simulink model "Gaussian_Distribution_validation"  (R2024a)
settings: Solver=VariableStepAuto  StartTime=0.0  StopTime=0.005  RelTol=1e-3
libraries: hdlBasic x26, vmcUtilities x1
settings Model: Creator=ehtisham  LastModifiedBy=ehtisham

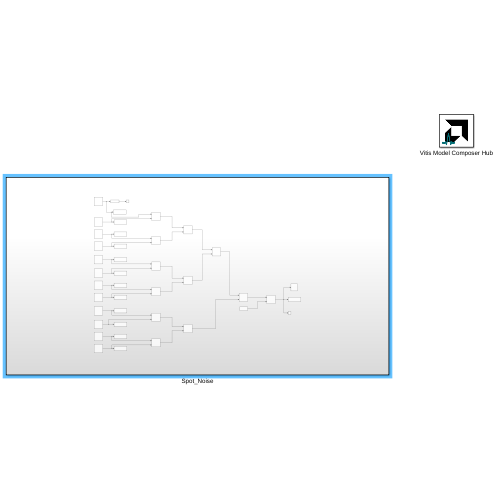
[thumbnail: Simulink's stored preview of the top-level diagram]
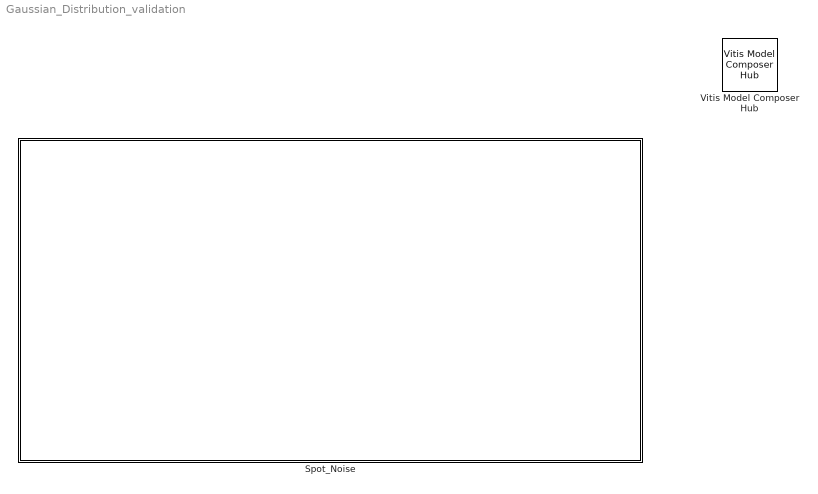
== system Gaussian_Distribution_validation ==
  Spot_Noise : Subsystem
  Vitis Model Composer Hub : vmcUtilities/Vitis Model Composer Hub  Tag=genX  CodeGeneration=off  SubsystemName=Spot_Noise  CompilationType=HDLCompilation  ExportTypeV2=IP Catalog  StartColumn=1  NumberOfColumns=1  TargetDirectory=./netlist  exportDesign=off  analyzeDesign=off  validateDesignOnHw=off  ExportType=AI Engines  IpVendor=xilinx.com  IpLibrary=hls  IpVersion=1.0  IpHWLanguage=Verilog  AieCompilerOptions={}  AieSimulatorOptions={}  CreateTestbench=off  TestbenchStackSize=10  RunRtlSim=off  RunCSim=off  RunAieSim=off  AieSimTimeout=50000  RunAieSimProfiling=off  LaunchVitisAnalyzer=off  PlotOutput=off  RunX86Sim=off  X86SimTimeout=10  GenHwImage=off  GenLibadfXo=on  GenHwValidationCode=off  PlatformType=Not Specified  HwSystemType=Baremetal  HwValidationTarget=hw  ProjDevice=Zynq UltraScale+ ZCU102 Evaluation Board (xczu9eg-ffvb1156-2-e)  ProjDevicePart=xczu9eg-ffvb1156-2-e  AIEType=None  SamplePeriod=-1  ClockFrequency=200  DataPathParallelism=1  xilinxfamily=zynquplus  part=xczu9eg  speed=-2-e  package=ffvb1156  directory=./netlist/ip/Spot_Noise/src  testbench=off  incr_netlist=off  synthesis_tool=Vivado  clock_wrapper=Clock Enables  dbl_ovrd=According to Block Masks  dcm_input_clock_period=10  sysclk_period=4  simulink_period=1/245760000  eval_field=0  LogFileName=''  NThreads=4

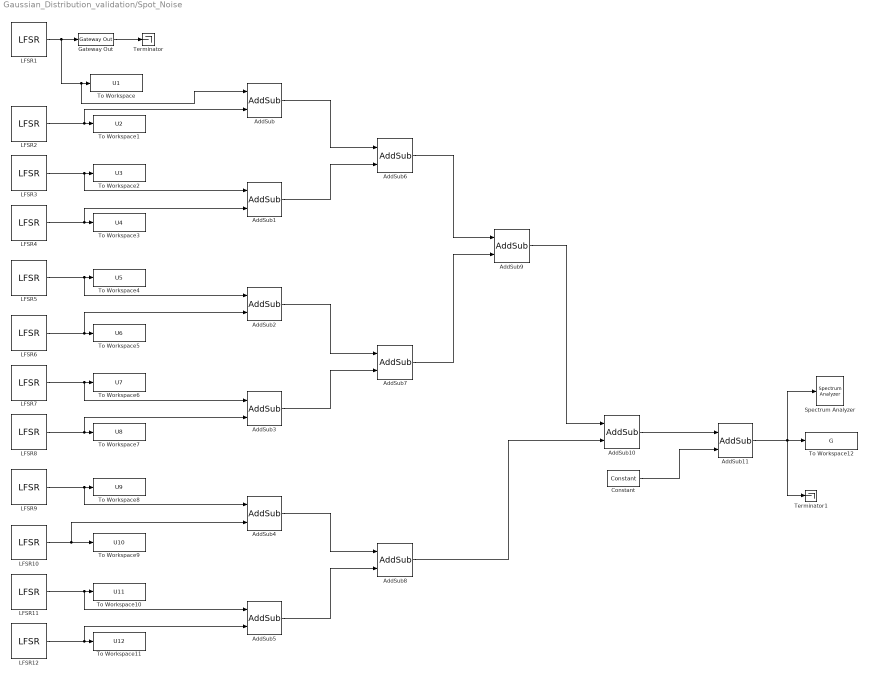
== system Gaussian_Distribution_validation/Spot_Noise ==
  AddSub{,1..10} (11 alike) : hdlBasic/AddSub  mode=Addition  use_carryin=off  use_carryout=off  en=off  latency=0  precision=Full  arith_type=Unsigned  n_bits=16  bin_pt=14  quantization=Truncate  overflow=Wrap  use_behavioral_HDL=off  hw_selection=Fabric  pipelined=off  XmcBlockStatus=1  maskContainerNames=tabcontainer1  block_type=addsub  block_config=sysgen:Addsub_config
  AddSub11 : hdlBasic/AddSub  mode=Subtraction  use_carryin=off  use_carryout=off  en=off  latency=0  precision=Full  arith_type=Unsigned  n_bits=16  bin_pt=14  quantization=Truncate  overflow=Wrap  use_behavioral_HDL=off  hw_selection=Fabric  pipelined=off  XmcBlockStatus=1  maskContainerNames=tabcontainer1  block_type=addsub  block_config=sysgen:Addsub_config
  Constant : hdlBasic/Constant  const=6  gui_display_data_type=Fixed-point  arith_type=Unsigned  n_bits=3  bin_pt=0  preci_type=Single  exp_width=8  frac_width=24  explicit_period=off  period=1  XmcBlockStatus=1  maskContainerNames=tabcontainer1  block_type=constant  block_config=sysgen:Constant_config
  Gateway Out : hdlBasic/Gateway Out  inherit_from_input=off  hdl_port=on  rows=1  columns=1  UseAsDAC=off  DACChannel='1'  interface=None  automatic_assignment=on  address_offset=hex2dec('00')  intf_name=''  intf_description=''  timing_constraint=None  locs_specified=off  LOCs={}  io_standard={}  XmcBlockStatus=1  maskContainerNames=group4  block_type=gatewayout  block_config=sysgen:gateway_out_config  block_width_w=590  block_height_w=620  block_width=620  block_height=750
  LFSR1 : hdlBasic/LFSR  lfsr_type=Fibonacci  gate_type=XNOR  n_bits=16  maxpolynomial=off  polynomial='2D'  rst_value='1'  rst=off  en=off  reloadable_seed=off  input_type=off  output_type=on  arith_type=Unsigned  bin_pt=16  explicit_period=on  period=1/245760000  XmcBlockStatus=1  maskContainerNames=tabcontainer1  block_type=lfsr  block_config=sysgen:LFSR_config
  LFSR10 : hdlBasic/LFSR  lfsr_type=Fibonacci  gate_type=XNOR  n_bits=16  maxpolynomial=off  polynomial='15D'  rst_value='1'  rst=off  en=off  reloadable_seed=off  input_type=off  output_type=on  arith_type=Unsigned  bin_pt=16  explicit_period=on  period=1/245760000  XmcBlockStatus=1  maskContainerNames=tabcontainer1  block_type=lfsr  block_config=sysgen:LFSR_config
  LFSR11 : hdlBasic/LFSR  lfsr_type=Fibonacci  gate_type=XNOR  n_bits=16  maxpolynomial=off  polynomial='197'  rst_value='1'  rst=off  en=off  reloadable_seed=off  input_type=off  output_type=on  arith_type=Unsigned  bin_pt=16  explicit_period=on  period=1/245760000  XmcBlockStatus=1  maskContainerNames=tabcontainer1  block_type=lfsr  block_config=sysgen:LFSR_config
  LFSR12 : hdlBasic/LFSR  lfsr_type=Fibonacci  gate_type=XNOR  n_bits=16  maxpolynomial=off  polynomial='1A1'  rst_value='1'  rst=off  en=off  reloadable_seed=off  input_type=off  output_type=on  arith_type=Unsigned  bin_pt=16  explicit_period=on  period=1/245760000  XmcBlockStatus=1  maskContainerNames=tabcontainer1  block_type=lfsr  block_config=sysgen:LFSR_config
  LFSR2 : hdlBasic/LFSR  lfsr_type=Fibonacci  gate_type=XNOR  n_bits=16  maxpolynomial=off  polynomial='39'  rst_value='1'  rst=off  en=off  reloadable_seed=off  input_type=off  output_type=on  arith_type=Unsigned  bin_pt=16  explicit_period=on  period=1/245760000  XmcBlockStatus=1  maskContainerNames=tabcontainer1  block_type=lfsr  block_config=sysgen:LFSR_config
  LFSR3 : hdlBasic/LFSR  lfsr_type=Fibonacci  gate_type=XNOR  n_bits=16  maxpolynomial=off  polynomial='3F'  rst_value='1'  rst=off  en=off  reloadable_seed=off  input_type=off  output_type=on  arith_type=Unsigned  bin_pt=16  explicit_period=on  period=1/245760000  XmcBlockStatus=1  maskContainerNames=tabcontainer1  block_type=lfsr  block_config=sysgen:LFSR_config
  LFSR4 : hdlBasic/LFSR  lfsr_type=Fibonacci  gate_type=XNOR  n_bits=16  maxpolynomial=off  polynomial='53'  rst_value='1'  rst=off  en=off  reloadable_seed=off  input_type=off  output_type=on  arith_type=Unsigned  bin_pt=16  explicit_period=on  period=1/245760000  XmcBlockStatus=1  maskContainerNames=tabcontainer1  block_type=lfsr  block_config=sysgen:LFSR_config
  LFSR5 : hdlBasic/LFSR  lfsr_type=Fibonacci  gate_type=XNOR  n_bits=16  maxpolynomial=off  polynomial='BD'  rst_value='1'  rst=off  en=off  reloadable_seed=off  input_type=off  output_type=on  arith_type=Unsigned  bin_pt=16  explicit_period=on  period=1/245760000  XmcBlockStatus=1  maskContainerNames=tabcontainer1  block_type=lfsr  block_config=sysgen:LFSR_config
  LFSR6 : hdlBasic/LFSR  lfsr_type=Fibonacci  gate_type=XNOR  n_bits=16  maxpolynomial=off  polynomial='D7'  rst_value='1'  rst=off  en=off  reloadable_seed=off  input_type=off  output_type=on  arith_type=Unsigned  bin_pt=16  explicit_period=on  period=1/245760000  XmcBlockStatus=1  maskContainerNames=tabcontainer1  block_type=lfsr  block_config=sysgen:LFSR_config
  LFSR7 : hdlBasic/LFSR  lfsr_type=Fibonacci  gate_type=XNOR  n_bits=16  maxpolynomial=off  polynomial='12F'  rst_value='1'  rst=off  en=off  reloadable_seed=off  input_type=off  output_type=on  arith_type=Unsigned  bin_pt=16  explicit_period=on  period=1/245760000  XmcBlockStatus=1  maskContainerNames=tabcontainer1  block_type=lfsr  block_config=sysgen:LFSR_config
  LFSR8 : hdlBasic/LFSR  lfsr_type=Fibonacci  gate_type=XNOR  n_bits=16  maxpolynomial=off  polynomial='13D'  rst_value='1'  rst=off  en=off  reloadable_seed=off  input_type=off  output_type=on  arith_type=Unsigned  bin_pt=16  explicit_period=on  period=1/245760000  XmcBlockStatus=1  maskContainerNames=tabcontainer1  block_type=lfsr  block_config=sysgen:LFSR_config
  LFSR9 : hdlBasic/LFSR  lfsr_type=Fibonacci  gate_type=XNOR  n_bits=16  maxpolynomial=off  polynomial='14F'  rst_value='1'  rst=off  en=off  reloadable_seed=off  input_type=off  output_type=on  arith_type=Unsigned  bin_pt=16  explicit_period=on  period=1/245760000  XmcBlockStatus=1  maskContainerNames=tabcontainer1  block_type=lfsr  block_config=sysgen:LFSR_config
  Spectrum Analyzer : SpectrumAnalyzer  WindowPosition=[365.000000,160.000000,800.000000,500.000000,]  ScopeFrameLocation=window  Span=245760000  StartFrequency=-122880000  StopFrequency=122880000  YLimits=[-9.5999377,7.8120668]
  Terminator : Terminator
  Terminator1 : Terminator
  To Workspace : ToWorkspace  VariableName=U1  SaveFormat=Timeseries  SampleTime=-1
  To Workspace1 : ToWorkspace  VariableName=U2  SaveFormat=Timeseries  SampleTime=-1
  To Workspace10 : ToWorkspace  VariableName=U11  SaveFormat=Timeseries  SampleTime=-1
  To Workspace11 : ToWorkspace  VariableName=U12  SaveFormat=Timeseries  SampleTime=-1
  To Workspace12 : ToWorkspace  VariableName=G  SaveFormat=Timeseries  SampleTime=-1
  To Workspace2 : ToWorkspace  VariableName=U3  SaveFormat=Timeseries  SampleTime=-1
  To Workspace3 : ToWorkspace  VariableName=U4  SaveFormat=Timeseries  SampleTime=-1
  To Workspace4 : ToWorkspace  VariableName=U5  SaveFormat=Timeseries  SampleTime=-1
  To Workspace5 : ToWorkspace  VariableName=U6  SaveFormat=Timeseries  SampleTime=-1
  To Workspace6 : ToWorkspace  VariableName=U7  SaveFormat=Timeseries  SampleTime=-1
  To Workspace7 : ToWorkspace  VariableName=U8  SaveFormat=Timeseries  SampleTime=-1
  To Workspace8 : ToWorkspace  VariableName=U9  SaveFormat=Timeseries  SampleTime=-1
  To Workspace9 : ToWorkspace  VariableName=U10  SaveFormat=Timeseries  SampleTime=-1
  wires:
  LFSR1/1 -> Gateway Out/1, AddSub/1, To Workspace/1
  Gateway Out/1 -> Terminator/1
  LFSR2/1 -> AddSub/2, To Workspace1/1
  LFSR3/1 -> AddSub1/1, To Workspace2/1
  LFSR4/1 -> AddSub1/2, To Workspace3/1
  LFSR5/1 -> AddSub2/1, To Workspace4/1
  LFSR9/1 -> AddSub4/1, To Workspace8/1
  LFSR8/1 -> AddSub3/2, To Workspace7/1
  LFSR7/1 -> AddSub3/1, To Workspace6/1
  LFSR6/1 -> AddSub2/2, To Workspace5/1
  LFSR10/1 -> AddSub4/2, To Workspace9/1
  LFSR11/1 -> AddSub5/1, To Workspace10/1
  LFSR12/1 -> AddSub5/2, To Workspace11/1
  AddSub/1 -> AddSub6/1
  AddSub1/1 -> AddSub6/2
  AddSub2/1 -> AddSub7/1
  AddSub3/1 -> AddSub7/2
  AddSub4/1 -> AddSub8/1
  AddSub5/1 -> AddSub8/2
  AddSub6/1 -> AddSub9/1
  AddSub7/1 -> AddSub9/2
  AddSub9/1 -> AddSub10/1
  AddSub8/1 -> AddSub10/2
  Constant/1 -> AddSub11/2
  AddSub10/1 -> AddSub11/1
  AddSub11/1 -> Terminator1/1, Spectrum Analyzer/1, To Workspace12/1
